simulink model "double_integrator_pd"  (R2020b)
settings: Solver=VariableStepAuto  StartTime=0.0  StopTime=10.0  RelTol=1e-3
values from neighbouring files (symbols this model uses):
  Current_coordinates = [Prev_Px(i); Prev_Py(i)]    [lloyd_wtd_heterogeneous.m]    (also in lloyd_wtd_heterogeneous_adaptive.m)
  Target_coordinates = [Px(i);Py(i)]    [lloyd_wtd_heterogeneous.m]    (also in lloyd_wtd_heterogeneous_adaptive.m)
libraries: simulink x1
settings Model: Creator=nijil  LastModifiedBy=nijil

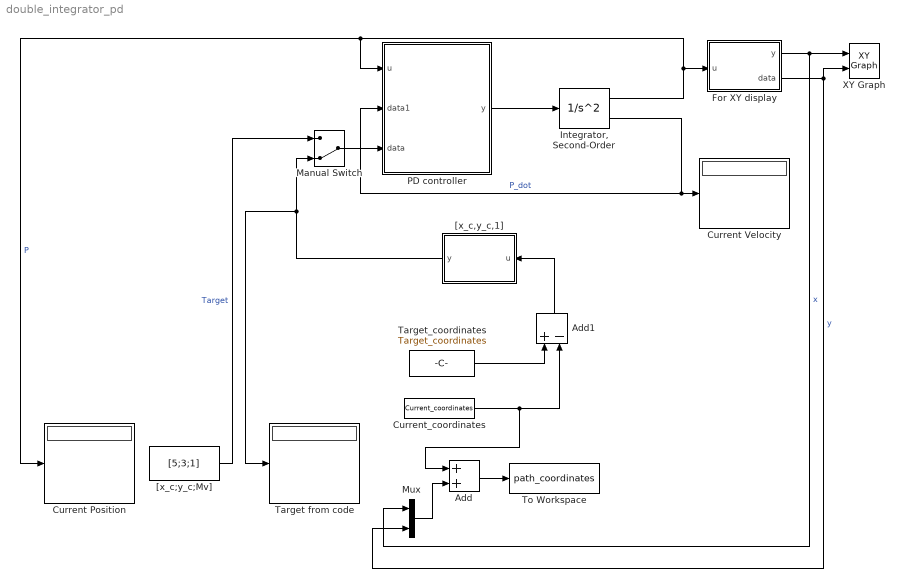
== system double_integrator_pd ==
  Add : Sum
  Add1 : Sum  Inputs=+-
  Current Position : Display
  Current Velocity : Display
  Current_coordinates : Constant  Value=Current_coordinates
  For XY display : MATLAB Function  TreatAsAtomicUnit=on
  "Integrator, Second-Order" : SecondOrderIntegrator
  Manual Switch : ManualSwitch  CurrentSetting=0
  Mux : Mux  Inputs=2
  PD controller : MATLAB Function  TreatAsAtomicUnit=on
  Target from code : Display
  Target_coordinates : Constant  Value=Target_coordinates
  To Workspace : ToWorkspace  VariableName=path_coordinates  SaveFormat=Timeseries  SampleTime=-1
  XY Graph : simulink/Sinks/XY Graph  xmin=-10  xmax=10  ymin=-10  ymax=10  st=-1
  "[x_c,y_c,1]" : MATLAB Function  TreatAsAtomicUnit=on
  "[x_c;y_c;Mv]" : Constant  Value=[5;3;1]
  wires:
  PD controller/1(y) -> "Integrator, Second-Order"/1
  "Integrator, Second-Order"/1 -> PD controller/1(u), Current Position/1, For XY display/1(u)  "P"
  For XY display/1(y) -> Mux/1, XY Graph/1  "x"
  For XY display/2(data) -> Mux/2, XY Graph/2  "y"
  "Integrator, Second-Order"/2 -> PD controller/2(data1), Current Velocity/1  "P_dot"
  Mux/1 -> Add/2
  Target_coordinates/1 -> Add1/1
  Add1/1 -> "[x_c,y_c,1]"/1(u)
  Current_coordinates/1 -> Add1/2, Add/1
  Add/1 -> To Workspace/1
  "[x_c,y_c,1]"/1(y) -> Target from code/1, Manual Switch/2
  "[x_c;y_c;Mv]"/1 -> Manual Switch/1  "Target"
  Manual Switch/1 -> PD controller/3(data)

== matlab function double_integrator_pd/PD controller ==
  data: u input; data1 input; y output; data input
function y = fcn(u, data1, data)
%data=[x_c;y_c;M_v] u=[x;y] data1=[x_dot;y_dot]
k1=3;
k2=2;
Cv=data(1:2);
y = -k1*data(3)*(u-Cv)-k2*data1;

== matlab function double_integrator_pd/For XY display ==
  data: u input; y output; data output
function [y,data] = fcn(u)
y=u(1);
data = u(2);

== matlab function double_integrator_pd/[x_c,y_c,1] ==
  data: u input; y output
function y = fcn(u)

y = [u(1),u(2),1];
